simulink model "brightnessController"  (R2020b)
settings: Solver=VariableStepAuto  StartTime=0.0  StopTime=10.0  RelTol=1e-3
settings Model: Creator=Balazs  LastModifiedBy=Balazs

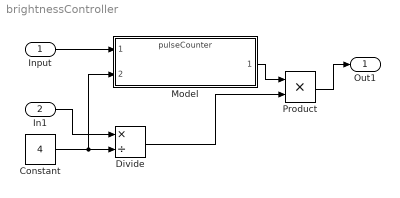
== system brightnessController ==
  Input : Inport  OutDataTypeStr=boolean
  In1 : Inport  Port=2  OutDataTypeStr=uint16
  Constant : Constant  Value=4  OutDataTypeStr=uint8
  Divide : Product  Inputs=*/  OutDataTypeStr=uint16
  Model : ModelReference  ModelNameDialog=pulseCounter.slx  SimulationMode=Normal  ModelReferenceVersion=1.15
  Product : Product  OutDataTypeStr=uint16
  Out1 : Outport  OutDataTypeStr=uint16
  wires:
  Input/1 -> Model/1
  Constant/1 -> Divide/2, Model/2
  Model/1 -> Product/1
  Product/1 -> Out1/1
  In1/1 -> Divide/1
  Divide/1 -> Product/2
